simulink model "Simulink_Simulation"  (R2022b)
settings: Solver=FixedStepAuto  StartTime=0.0  StopTime=20  FixedStep=5e-4  RelTol=1e-3
values from neighbouring files (symbols this model uses):
  Kd_PitchRate1 = MPar(3)    [PID_Pitch_Evaluation.m]    (also in PID_Pitch_Evaluation_func.m; PID_Simulation_Init.m = -20)
  Kd_PitchRate2 = -0    (= 0)    [PID_Pitch_Evaluation.m]    (also in PID_Simulation_Init.m)
  Ki_PitchRate1 = MPar(2)    [PID_Pitch_Evaluation.m]    (also in PID_Pitch_Evaluation_func.m; PID_Simulation_Init.m = -20)
  Ki_PitchRate2 = -0    (= 0)    [PID_Pitch_Evaluation.m]    (also in PID_Simulation_Init.m)
  Kp_PitchRate1 = MPar(1)    [PID_Pitch_Evaluation.m]    (also in PID_Pitch_Evaluation_func.m; PID_Simulation_Init.m = -50)
  Kp_PitchRate2 = -0    (= 0)    [PID_Pitch_Evaluation.m]    (also in PID_Simulation_Init.m)
  m = 1.172    [Transfer_Functions_Simplified.m]
  N_PitchRate1 = MPar(4)    [PID_Pitch_Evaluation.m]    (also in PID_Pitch_Evaluation_func.m; PID_Simulation_Init.m = 10)
  N_PitchRate2 = 5    [PID_Pitch_Evaluation.m]    (also in PID_Simulation_Init.m = 4)
  Ts = 0.005    [PID_Pitch_Evaluation.m]    (also in PID_Pitch_Evaluation_func.m; PID_Simulation_Init.m = 0.01)
undefined symbols (not defined in the file or in its folder): DiscIntNeverNeededParam, smiData, X, Y, Z
libraries: sm_lib x25, nesl_utility x14, slpidlib x6, simulink x1
(part 2 of 2)

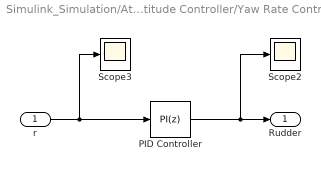
== system Simulink_Simulation/Attitude Controller/Yaw Rate Controller ==
  r : Inport
  PID Controller : slpidlib/PID Controller  Controller=PI  Form=Parallel  TimeDomain=Discrete-time  UseExternalTs=off  SampleTime=0.01  IntegratorMethod=Forward Euler  FilterMethod=Forward Euler  ControllerParametersSource=internal  P=1261751  I=255231  UseKiTs=off  D=10000  N=0.5  UseFilter=on  TunerSelectOption=Transfer Function Based (PID Tuner App)  InitialConditionSource=internal  InitialConditionForIntegrator=0  InitialConditionForFilter=0  DifferentiatorICPrevScaledInput=0  ExternalReset=none  TrackingMode=off  Kt=1  LimitOutput=off  SatLimitsSource=internal  UpperSaturationLimit=inf  LowerSaturationLimit=-inf  LinearizeAsGain=on  AntiWindupMode=none  Kb=1  LimitIntegrator=off  UpperIntegratorSaturationLimit=inf  LowerIntegratorSaturationLimit=-inf  POutMin=[]  POutMax=[]  IOutMin=[]  IOutMax=[]  DOutMin=[]  DOutMax=[]  NOutMin=[]  NOutMax=[]  SumOutMin=[]  SumOutMax=[]  SaturationOutMin=[]  SaturationOutMax=[]  PParamMin=[]  PParamMax=[]  IParamMin=[]  IParamMax=[]  DParamMin=[]  DParamMax=[]  NParamMin=[]  NParamMax=[]  KbParamMin=[]  KbParamMax=[]  KtParamMin=[]  KtParamMax=[]  KbOutMin=[]  KbOutMax=[]  KtOutMin=[]  KtOutMax=[]  IntegratorOutMin=[]  IntegratorOutMax=[]  FilterOutMin=[]  FilterOutMax=[]  SumI1OutMin=[]  SumI1OutMax=[]  SumI2OutMin=[]  SumI2OutMax=[]  SumI3OutMin=[]  SumI3OutMax=[]  SumI4OutMin=[]  SumI4OutMax=[]  SumDOutMin=[]  SumDOutMax=[]  DifferentiatorOutMin=[]  DifferentiatorOutMax=[]  FilterDiffOutCoefMin=[]  FilterDiffOutCoefMax=[]  ReciprocalOutMin=[]  ReciprocalOutMax=[]  SumDenOutMin=[]  SumDenOutMax=[]  SumNumOutMin=[]  SumNumOutMax=[]  DivideOutMin=[]  DivideOutMax=[]  UdiffTsProdOutMin=[]  UdiffTsProdOutMax=[]  NTsProdOutMin=[]  NTsProdOutMax=[]  UintegralTsProdOutMin=[]  UintegralTsProdOutMax=[]  UngainTsProdOutMin=[]  UngainTsProdOutMax=[]  ClampingZeroOutDataTypeStr=Inherit: Inherit via back propagation  ClampingZeroOutMin=[]  ClampingZeroOutMax=[]  FilterDenConstantOutDataTypeStr=Inherit: Inherit via back propagation  FilterDenConstantOutMin=[]  FilterDenConstantOutMax=[]  PCopyOutDataTypeStr=Inherit: Inherit via back propagation  PCopyOutMin=[]  PCopyOutMax=[]  NCopyOutDataTypeStr=Inherit: Inherit via back propagation  NCopyOutMin=[]  NCopyOutMax=[]  IntegratorContinuousStateAttributes=''  IntegratorStateMustResolveToSignalObject=off  IntegratorRTWStateStorageClass=Auto  FilterContinuousStateAttributes=''  FilterStateMustResolveToSignalObject=off  FilterRTWStateStorageClass=Auto  ParallelPVariant=InternalParameters  IdealPVariant=Disabled  IVariant=InternalParameters  DVariant=Disabled  IntegratorVariant=Discrete  SatVariant=Disabled  AWVariant=Passthrough  PCopyVariant=Disabled  TRVariant=Disabled  FdbkBlocksVariant=Forward  IdealPFdbkVariant=Disabled  SatFdbkVariant=Disabled  DerivativeFilterVariant=Disabled  NVariant=Disabled  NCopyVariant=Disabled_SignalSpec  FilterICVariant=Disabled  IntegratorICVariant=InternalICs  ExternalResetVariant=Disabled  TRSumVariant=Passthrough  SumFdbkVariant=Disabled  SumVariant=Sum_PI  TsampFilterVariant=InternalTs  TsampNgainVariant=Passthrough  TsampIntegralVariant=Passthrough  ExternalSaturationOutDataTypeStr=Inherit: Same as second input
  Scope2 : Scope
  Scope3 : Scope
  Rudder : Outport
  wires:
  PID Controller/1 -> Scope2/1, Rudder/1
  r/1 -> Scope3/1, PID Controller/1

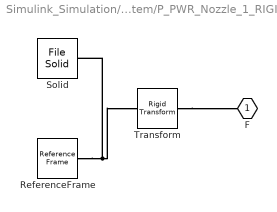
== system Simulink_Simulation/Aircraft Dynamics/Subsystem/P_PWR_Nozzle_1_RIGID ==
  ReferenceFrame : sm_lib/Frames and Transforms/Reference Frame
  Solid : sm_lib/Body Elements/File Solid  ExtGeomFileName=#P_PWR_Nozzle_Predeterminado_sldprt.STEP  UnitType=FromFile  ExtGeomFileUnits=m  StepReaderType=HEX  ExportConvexHullGeometry=off  InertiaType=Custom  Mass=smiData.Solid(2).mass  MassUnits=kg  CenterOfMass=smiData.Solid(2).CoM  CenterOfMassUnits=mm  MomentsOfInertia=smiData.Solid(2).MoI  MomentsOfInertiaUnits=kg*mm^2  ProductsOfInertia=smiData.Solid(2).PoI  ProductsOfInertiaUnits=kg*mm^2  BasedOnType=DensityFromFile  Density=1000  DensityUnits=kg/m^3  DoExposeReferenceFrame=on  SerializedFrames=<Frames/>  GraphicType=FromGeometry  MarkerShape=Sphere  MarkerSize=10  GraphicVisPropType=SimpleVisualProperties  GraphicDiffuseColor=smiData.Solid(2).color  GraphicSpecularColor=[0.5 0.5 0.5 1.0]  GraphicAmbientColor=[0.15 0.15 0.15 1.0]  GraphicEmissiveColor=[0.0 0.0 0.0 1.0]  GraphicShininess=75  GraphicOpacity=smiData.Solid(2).opacity
  Transform : sm_lib/Frames and Transforms/Rigid Transform  TranslationMethod=Cartesian  TranslationStandardOffset=0  TranslationLengthUnit=mm  TranslationStandardAxis=+Z  TranslationCartesianOffset=smiData.RigidTransform(2).translation  TranslationROffset=0  TranslationROffsetUnits=m  TranslationZOffset=0  TranslationZOffsetUnits=m  TranslationThetaOffset=0  TranslationThetaOffsetUnits=deg  RotationMethod=ArbitraryAxis  RotationAngleUnits=rad  RotationStandardAxis=+Z  RotationAngle=smiData.RigidTransform(2).angle  RotationArbitraryAxis=smiData.RigidTransform(2).axis  FollAlignAxisA=+X  BaseAlignAxisA=+Y  FollAlignAxisB=+Y  BaseAlignAxisB=+Z  RotationSequenceAxes=FollowerAxes  RotationSequence=XYX  RotationSequenceAngles=[0 0 0]  RotationSequenceAnglesUnits=deg  RotationMatrix=[1 0 0; 0 1 0; 0 0 1]  Quaternion=[1 0 0 0]
  F : PMIOPort  Side=Left
  connections:
  Solid/RConn1 -- ReferenceFrame/RConn1 -- Transform/LConn1
  Transform/RConn1 -- F/RConn1

== system Simulink_Simulation/Aircraft Dynamics/Subsystem/P_PWR_Nozzle_2_RIGID ==
  ReferenceFrame : sm_lib/Frames and Transforms/Reference Frame
  Solid : sm_lib/Body Elements/File Solid  ExtGeomFileName=#P_PWR_Nozzle_Predeterminado_sldprt.STEP  UnitType=FromFile  ExtGeomFileUnits=m  StepReaderType=HEX  ExportConvexHullGeometry=off  InertiaType=Custom  Mass=smiData.Solid(2).mass  MassUnits=kg  CenterOfMass=smiData.Solid(2).CoM  CenterOfMassUnits=mm  MomentsOfInertia=smiData.Solid(2).MoI  MomentsOfInertiaUnits=kg*mm^2  ProductsOfInertia=smiData.Solid(2).PoI  ProductsOfInertiaUnits=kg*mm^2  BasedOnType=DensityFromFile  Density=1000  DensityUnits=kg/m^3  DoExposeReferenceFrame=on  SerializedFrames=<Frames/>  GraphicType=FromGeometry  MarkerShape=Sphere  MarkerSize=10  GraphicVisPropType=SimpleVisualProperties  GraphicDiffuseColor=smiData.Solid(2).color  GraphicSpecularColor=[0.5 0.5 0.5 1.0]  GraphicAmbientColor=[0.15 0.15 0.15 1.0]  GraphicEmissiveColor=[0.0 0.0 0.0 1.0]  GraphicShininess=75  GraphicOpacity=smiData.Solid(2).opacity
  Transform : sm_lib/Frames and Transforms/Rigid Transform  TranslationMethod=Cartesian  TranslationStandardOffset=0  TranslationLengthUnit=mm  TranslationStandardAxis=+Z  TranslationCartesianOffset=smiData.RigidTransform(4).translation  TranslationROffset=0  TranslationROffsetUnits=m  TranslationZOffset=0  TranslationZOffsetUnits=m  TranslationThetaOffset=0  TranslationThetaOffsetUnits=deg  RotationMethod=ArbitraryAxis  RotationAngleUnits=rad  RotationStandardAxis=+Z  RotationAngle=smiData.RigidTransform(4).angle  RotationArbitraryAxis=smiData.RigidTransform(4).axis  FollAlignAxisA=+X  BaseAlignAxisA=+Y  FollAlignAxisB=+Y  BaseAlignAxisB=+Z  RotationSequenceAxes=FollowerAxes  RotationSequence=XYX  RotationSequenceAngles=[0 0 0]  RotationSequenceAnglesUnits=deg  RotationMatrix=[1 0 0; 0 1 0; 0 0 1]  Quaternion=[1 0 0 0]
  F : PMIOPort  Side=Left
  connections:
  Solid/RConn1 -- ReferenceFrame/RConn1 -- Transform/LConn1
  Transform/RConn1 -- F/RConn1

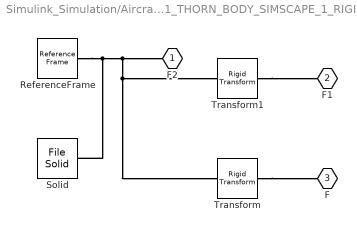
== system Simulink_Simulation/Aircraft Dynamics/Subsystem/X1_THORN_BODY_SIMSCAPE_1_RIGID ==
  ReferenceFrame : sm_lib/Frames and Transforms/Reference Frame
  Solid : sm_lib/Body Elements/File Solid  ExtGeomFileName=X1_THORN_BODY_SIMSCAPE_Predeterminado_sldprt.STEP  UnitType=FromFile  ExtGeomFileUnits=m  StepReaderType=HEX  ExportConvexHullGeometry=off  InertiaType=Custom  Mass=1021.99  MassUnits=g  CenterOfMass=[0, 0, 0]  CenterOfMassUnits=mm  MomentsOfInertia=[2841.18, 3338.08, 5733.93]  MomentsOfInertiaUnits=kg*mm^2  ProductsOfInertia=[0,0,0]  ProductsOfInertiaUnits=kg*mm^2  BasedOnType=DensityFromFile  Density=1000  DensityUnits=kg/m^3  DoExposeReferenceFrame=on  SerializedFrames=<Frames/>  GraphicType=FromGeometry  MarkerShape=Sphere  MarkerSize=10  GraphicVisPropType=SimpleVisualProperties  GraphicDiffuseColor=smiData.Solid(1).color  GraphicSpecularColor=[0.5 0.5 0.5 1.0]  GraphicAmbientColor=[0.15 0.15 0.15 1.0]  GraphicEmissiveColor=[0.0 0.0 0.0 1.0]  GraphicShininess=75  GraphicOpacity=smiData.Solid(1).opacity
  Transform : sm_lib/Frames and Transforms/Rigid Transform  TranslationMethod=Cartesian  TranslationStandardOffset=0  TranslationLengthUnit=mm  TranslationStandardAxis=+Z  TranslationCartesianOffset=smiData.RigidTransform(1).translation  TranslationROffset=0  TranslationROffsetUnits=m  TranslationZOffset=0  TranslationZOffsetUnits=m  TranslationThetaOffset=0  TranslationThetaOffsetUnits=deg  RotationMethod=ArbitraryAxis  RotationAngleUnits=rad  RotationStandardAxis=+Z  RotationAngle=smiData.RigidTransform(1).angle  RotationArbitraryAxis=smiData.RigidTransform(1).axis  FollAlignAxisA=+X  BaseAlignAxisA=+Y  FollAlignAxisB=+Y  BaseAlignAxisB=+Z  RotationSequenceAxes=FollowerAxes  RotationSequence=XYX  RotationSequenceAngles=[0 0 0]  RotationSequenceAnglesUnits=deg  RotationMatrix=[1 0 0; 0 1 0; 0 0 1]  Quaternion=[1 0 0 0]
  Transform1 : sm_lib/Frames and Transforms/Rigid Transform  TranslationMethod=Cartesian  TranslationStandardOffset=0  TranslationLengthUnit=mm  TranslationStandardAxis=+Z  TranslationCartesianOffset=smiData.RigidTransform(3).translation  TranslationROffset=0  TranslationROffsetUnits=m  TranslationZOffset=0  TranslationZOffsetUnits=m  TranslationThetaOffset=0  TranslationThetaOffsetUnits=deg  RotationMethod=ArbitraryAxis  RotationAngleUnits=rad  RotationStandardAxis=+Z  RotationAngle=smiData.RigidTransform(3).angle  RotationArbitraryAxis=smiData.RigidTransform(3).axis  FollAlignAxisA=+X  BaseAlignAxisA=+Y  FollAlignAxisB=+Y  BaseAlignAxisB=+Z  RotationSequenceAxes=FollowerAxes  RotationSequence=XYX  RotationSequenceAngles=[0 0 0]  RotationSequenceAnglesUnits=deg  RotationMatrix=[1 0 0; 0 1 0; 0 0 1]  Quaternion=[1 0 0 0]
  F2 : PMIOPort  Side=Left
  F1 : PMIOPort  Port=2  Side=Right
  F : PMIOPort  Port=3  Side=Right
  connections:
  Solid/RConn1 -- ReferenceFrame/RConn1 -- Transform/LConn1 -- Transform1/LConn1 -- F2/RConn1
  Transform/RConn1 -- F/RConn1
  Transform1/RConn1 -- F1/RConn1

== matlab function Simulink_Simulation/Vertical Acceleration Controller/MATLAB Function ==
  data: omega input; omega1 input; omega1_PID output; omega2 input; omega2_PID output
function [omega1_PID, omega2_PID] = fcn(omega, omega1, omega2)



delta = (omega1-omega2)/2;

omega1_PID = omega + delta;
omega2_PID = omega - delta;

== matlab function Simulink_Simulation/Aircraft Dynamics/Thrust Vectoring Forces/MATLAB Function ==
  data: omega1 input; Tx_ctrl output; omega2 input; alfa1 input; alfa2 input; Ty_ctrl output; Tz_ctrl output; Mx_ctrl output; My_ctrl output; Mz_ctrl output
function [Tx_ctrl, Ty_ctrl, Tz_ctrl, Mx_ctrl, My_ctrl, Mz_ctrl] = fcn(omega1, omega2, alfa1, alfa2)

%% Compute Forces based on inputs

% Test Stand Constants

setpoint_R = 1600; % Servo setpoint (neutral 0 deg)
setpoint_L = 1600;

A_Tx = 3.45e-8;
B_Tx = 3e-3;

A_Tz = -1.0e-8;
B_Tz = 7e-3;

A_My = -1.3e-12;
B_My = 8e-3;

% Thrust calculation

Tx_R = A_Tx*omega1^2*cos((alfa1-setpoint_R)*B_Tx);
Tz_R = A_Tz*omega1^2*sin((alfa1-setpoint_R)*B_Tz);
My_R = A_My*omega1^2*sin((alfa1-setpoint_R)*B_My);

Tx_L = A_Tx*omega2^2*cos((alfa2-setpoint_L)*B_Tx);
Tz_L = A_Tz*omega2^2*sin((alfa2-setpoint_L)*B_Tz);
My_L = A_My*omega2^2*sin((alfa2-setpoint_L)*B_My);

% Airframe parameters

x_CoG = 22.82e-3; % m
z_CoG = 0.35e-3; % m
lt_x = 60e-3; % m
lt_y = 72.5e-3; % m

% Control forces calculation

Tx_ctrl = Tx_R + Tx_L;
Ty_ctrl = 0;
Tz_ctrl = Tz_R - Tz_L;

Mx_ctrl = (Tz_R + Tz_L) * lt_y;
My_ctrl = My_R - My_L - (Tx_L + Tx_R) * z_CoG + (Tz_R * (x_CoG - lt_x)) - (Tz_L * (x_CoG - lt_x));
Mz_ctrl = (Tx_L - Tx_R) * lt_y;

== matlab function Simulink_Simulation/Attitude Controller/Reference Generator ==
  data: q0 input; p_error output; q1 input; q2 input; q3 input; pitch input; roll input; q_error output; r_error output
function [p_error,q_error,r_error] = fcn(q0, q1, q2, q3, pitch, roll)

q_curr = [q0;q1;q2;q3];

vec_x_Aircraft = [1-2*(q2^2+q3^2); 2*(q1*q2 + q0*q3); 2*(q1*q3 - q0*q2)];
vec_y_Aircraft = [2*(q1*q2 - q0*q3); 1 - 2*(q1^2 + q3^2); 2*(q2*q3 + q0*q1)];
vec_z_Aircraft = [2*(q1*q3 + q0*q2); 2*(q2*q3 - q0*q1); 1-2*(q1^2+q2^2)];

vec_x_World = [0;0;1];
vec_z_World = cross(vec_x_World,vec_y_Aircraft);
vec_y_World = cross(vec_z_World,vec_x_World);


%% 3) Build base rotation matrix R0 = [x_w, y_w, z_w]
R0 = [vec_x_World, vec_y_World, vec_z_World];

%% 4) Build small rotations about world-frame X then Y
Rx = [ 1,         0,          0;
       0, cos(-roll), -sin(-roll);
       0, sin(-roll),  cos(-roll)];
   
Ry = [ cos(pitch), 0, sin(pitch);
             0, 1,       0;
      -sin(pitch), 0, cos(pitch)];

% Composite: first roll (Rx), then pitch (Ry) in the *world frame*
R_ref = Rx * Ry * R0 ;

%% 5) Convert R_ref into quaternion [q0_ref q1_ref q2_ref q3_ref]
q_ref = rotm2quat(R_ref)';  % returns [w x y z]

if dot([q0,q1,q2,q3], q_ref) < 0

    q_ref = -q_ref;
end

% q0, q1 are 4×1 [q0; qv] quaternions (scalar-first)
dq = (q_ref - q_curr);

% build the 4×3 matrix M = [Ω(e1)q0, Ω(e2)q0, Ω(e3)q0]
e = eye(3);
M = zeros(4,3);
for i = 1:3
    M(:,i) = Omega(e(i,:)) * q_curr;
end

omega = 2*(M \ dq);   % least-squares if slightly overdetermined
p_error = omega(1);
q_error = omega(2);
r_error = omega(3);






function O = Omega(w)
    % returns the 4×4 Ω(w) matrix for quaternion kinematics
    p = w(1); q = w(2); r = w(3);
    O = [  0, -p, -q, -r;
           p,  0,  r, -q;
           q, -r,  0,  p;
           r,  q, -p,  0 ];
end

end

== matlab function Simulink_Simulation/Attitude Controller/MATLAB Function ==
  data: Aileron input; servo_R output; Elevator input; Rudder input; omegaR_prev input; omegaL_prev input; servo_L output; omega_R output; omega_L output
function [servo_R, servo_L, omega_R, omega_L] = fcn(Aileron, Elevator, Rudder, omegaR_prev, omegaL_prev)

omega_squared = omegaR_prev^2 + omegaL_prev^2;

if (omega_squared/2 - Rudder) < 0

    omega_R = 0;
else

    omega_R = sqrt(omega_squared/2 - Rudder);
end


if (omega_squared/2 + Rudder) < 0

    omega_L = 0;
else
    
    omega_L = sqrt(omega_squared/2 + Rudder);
end

servo_R = -Aileron - Elevator;
servo_L = -Aileron + Elevator;
